simulink model "Demo2"  (Simulink 6.5)
settings: Solver=ode45  StartTime=0.0  StopTime=10.0  RelTol=1e-3
settings Model: Creator=suarezjl  LastModifiedBy=suarezjl
settings DataIOCC: SignalLoggingName=sigsOut
settings DebuggingCC: SolverPrmCheckMsg=none  MultiTaskDSMMsg=warning  MultiTaskCondExecSysMsg=none  StrictBusMsg=None
settings HardwareCC: TargetUnknown=on
settings RTWCC: IncludeERTFirstTime=on

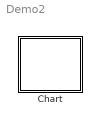
== system Demo2 ==
  Chart : Stateflow chart

== stateflow chart Chart ==
  state StartCameras
    \\Sally\HeadTrackingDemo\HeadModule\LeftCameraAgent\StateMachine.LoadSM()
    \\Sally\HeadTrackingDemo\HeadModule\LeftCameraAgent\StateMachine.Start()
    \\Sally\HeadTrackingDemo\HeadModule\RightCameraAgent\StateMachine.LoadSM()
    \\Sally\HeadTrackingDemo\HeadModule\RightCameraAgent\StateMachine.Start()
  state StartHead
    \\Sally\HeadTrackingDemo\HeadModule\HeadAgent\StateMachine.LoadSM()
    \\Sally\HeadTrackingDemo\HeadModule\HeadAgent\StateMachine.Start()
  state Stop
    \\Sally\HeadTrackingDemo\HeadModule\HeadAgent\StateMachine.Stop()
    \\Sally\HeadTrackingDemo\HeadModule\LeftCameraAgent\StateMachine.Stop()
    \\Sally\HeadTrackingDemo\HeadModule\RightCameraAgent\StateMachine.Stop()
  (default) -> StartCameras : Start
  StartCameras -> StartHead : Always
  StartHead -> Stop : Stop
